simulink model "Arm_Assembly"  (R2025b)
settings: Solver=ode23t  StartTime=0.0  StopTime=10.0  RelTol=1e-3
model workspace: external: MATLAB File C:\Users\kavin\Documents\MATLAB\Arm Project\Arm_Assembly_DataFile.m (data not in the file)
values from neighbouring files (symbols this model uses):
  s = dot(w, u)    [inverse_kinematics.m]
undefined symbols (not defined in the file or in its folder): smiData, X, Y, Z
libraries: sm_lib x36, nesl_utility x14, slpidlib x5
(part 2 of 2)

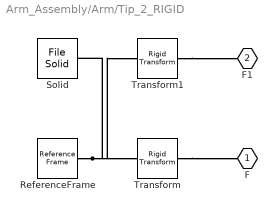
== system Arm_Assembly/Arm/Tip_2_RIGID ==
  ReferenceFrame : sm_lib/Frames and Transforms/Reference Frame
  Solid : sm_lib/Body Elements/File Solid  ExtGeomFileName=Tip_Default_sldprt.STEP  UnitType=FromFile  ExtGeomFileUnits=m  StepReaderType=HEX  ExportConvexHullGeometry=off  InertiaType=Custom  BasedOnType=DensityFromFile  Density=1000  DensityUnits=kg/m^3  Mass=smiData.Solid(7).mass  MassUnits=kg  CenterOfMass=smiData.Solid(7).CoM  CenterOfMassUnits=in  MomentsOfInertia=smiData.Solid(7).MoI  MomentsOfInertiaUnits=kg*in^2  ProductsOfInertia=smiData.Solid(7).PoI  ProductsOfInertiaUnits=kg*in^2  GraphicType=FromGeometry  MarkerShape=Sphere  MarkerSize=10  GraphicVisPropType=SimpleVisualProperties  GraphicDiffuseColor=smiData.Solid(7).color  GraphicOpacity=smiData.Solid(7).opacity  GraphicSpecularColor=[0.5 0.5 0.5 1.0]  GraphicAmbientColor=[0.15 0.15 0.15 1.0]  GraphicEmissiveColor=[0.0 0.0 0.0 1.0]  GraphicShininess=75  DoExposeReferenceFrame=on  SerializedFrames=<Frames/>
  Transform : sm_lib/Frames and Transforms/Rigid Transform  RotationMethod=ArbitraryAxis  FollAlignAxisA=+X  BaseAlignAxisA=+Y  FollAlignAxisB=+Y  BaseAlignAxisB=+Z  RotationStandardAxis=+Z  RotationAngle=smiData.RigidTransform(10).angle  RotationAngleUnits=rad  RotationArbitraryAxis=smiData.RigidTransform(10).axis  RotationSequenceAxes=FollowerAxes  RotationSequence=XYX  RotationSequenceAngles=[0 0 0]  RotationSequenceAnglesUnits=deg  RotationMatrix=[1 0 0;0 1 0;0 0 1]  Quaternion=[1 0 0 0]  TranslationMethod=Cartesian  TranslationCartesianOffset=smiData.RigidTransform(10).translation  TranslationCartesianOffsetUnits=in  TranslationStandardAxis=+Z  TranslationStandardOffset=0  TranslationStandardOffsetUnits=m  TranslationROffset=0  TranslationROffsetUnits=m  TranslationThetaOffset=0  TranslationThetaOffsetUnits=deg  TranslationZOffset=0  TranslationZOffsetUnits=m
  Transform1 : sm_lib/Frames and Transforms/Rigid Transform  RotationMethod=ArbitraryAxis  FollAlignAxisA=+X  BaseAlignAxisA=+Y  FollAlignAxisB=+Y  BaseAlignAxisB=+Z  RotationStandardAxis=+Z  RotationAngle=smiData.RigidTransform(11).angle  RotationAngleUnits=rad  RotationArbitraryAxis=smiData.RigidTransform(11).axis  RotationSequenceAxes=FollowerAxes  RotationSequence=XYX  RotationSequenceAngles=[0 0 0]  RotationSequenceAnglesUnits=deg  RotationMatrix=[1 0 0;0 1 0;0 0 1]  Quaternion=[1 0 0 0]  TranslationMethod=Cartesian  TranslationCartesianOffset=smiData.RigidTransform(11).translation  TranslationCartesianOffsetUnits=in  TranslationStandardAxis=+Z  TranslationStandardOffset=0  TranslationStandardOffsetUnits=m  TranslationROffset=0  TranslationROffsetUnits=m  TranslationThetaOffset=0  TranslationThetaOffsetUnits=deg  TranslationZOffset=0  TranslationZOffsetUnits=m
  F : PMIOPort  Side=Left
  F1 : PMIOPort  Port=2  Side=Right
  connections:
  Solid/RConn1 -- ReferenceFrame/RConn1 -- Transform/LConn1 -- Transform1/LConn1
  Transform/RConn1 -- F/RConn1
  Transform1/RConn1 -- F1/RConn1

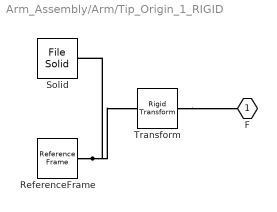
== system Arm_Assembly/Arm/Tip_Origin_1_RIGID ==
  ReferenceFrame : sm_lib/Frames and Transforms/Reference Frame
  Solid : sm_lib/Body Elements/File Solid  ExtGeomFileName=Tip_Origin_Default_sldprt.STEP  UnitType=FromFile  ExtGeomFileUnits=m  StepReaderType=HEX  ExportConvexHullGeometry=off  InertiaType=Custom  BasedOnType=DensityFromFile  Density=1000  DensityUnits=kg/m^3  Mass=smiData.Solid(1).mass  MassUnits=kg  CenterOfMass=smiData.Solid(1).CoM  CenterOfMassUnits=in  MomentsOfInertia=smiData.Solid(1).MoI  MomentsOfInertiaUnits=kg*in^2  ProductsOfInertia=smiData.Solid(1).PoI  ProductsOfInertiaUnits=kg*in^2  GraphicType=FromGeometry  MarkerShape=Sphere  MarkerSize=10  GraphicVisPropType=SimpleVisualProperties  GraphicDiffuseColor=smiData.Solid(1).color  GraphicOpacity=smiData.Solid(1).opacity  GraphicSpecularColor=[0.5 0.5 0.5 1.0]  GraphicAmbientColor=[0.15 0.15 0.15 1.0]  GraphicEmissiveColor=[0.0 0.0 0.0 1.0]  GraphicShininess=75  DoExposeReferenceFrame=on  SerializedFrames=<Frames/>
  Transform : sm_lib/Frames and Transforms/Rigid Transform  RotationMethod=ArbitraryAxis  FollAlignAxisA=+X  BaseAlignAxisA=+Y  FollAlignAxisB=+Y  BaseAlignAxisB=+Z  RotationStandardAxis=+Z  RotationAngle=smiData.RigidTransform(12).angle  RotationAngleUnits=rad  RotationArbitraryAxis=smiData.RigidTransform(12).axis  RotationSequenceAxes=FollowerAxes  RotationSequence=XYX  RotationSequenceAngles=[0 0 0]  RotationSequenceAnglesUnits=deg  RotationMatrix=[1 0 0;0 1 0;0 0 1]  Quaternion=[1 0 0 0]  TranslationMethod=Cartesian  TranslationCartesianOffset=smiData.RigidTransform(12).translation  TranslationCartesianOffsetUnits=in  TranslationStandardAxis=+Z  TranslationStandardOffset=0  TranslationStandardOffsetUnits=m  TranslationROffset=0  TranslationROffsetUnits=m  TranslationThetaOffset=0  TranslationThetaOffsetUnits=deg  TranslationZOffset=0  TranslationZOffsetUnits=m
  F : PMIOPort  Side=Left
  connections:
  Solid/RConn1 -- ReferenceFrame/RConn1 -- Transform/LConn1
  Transform/RConn1 -- F/RConn1

== matlab function Arm_Assembly/MATLAB Function ==
  data: x input; a1 output; y input; z input; r1 input; r2 input; a2 output; a3 output; a4 output; a5 output
function [a1, a2, a3, a4, a5] = inverse_kinematics(x, y, z, r1, r2)
    base = 1.25;
    L1 = 9.1601;
    L2 = 8.0463;
    L3 = 4.7889;
    L4 = 2.0304;
    tip = 2.5245;
    pos = [x, y, z];
    
    r1 = deg2rad(r1);
    r2 = deg2rad(r2);

    tip_v = [sin(r2)*cos(r1), cos(r2), sin(r2)*sin(r1)]; %direction of end
    A = tip_v * tip; %vector of end

    B = pos + A; %target of rest of body
   
    L3 = L3 + L4;
    a1 = atan2(B(3), B(1));
    a1 = a1 + pi - 0.1098;
    l1_v = [0, L1];

    B_t = [sqrt(B(1)*B(1) + B(3)*B(3)), B(2)]; %convert to 2d problem
    %l1 + L2 * <sin(a2), cos(a2)> + L3 * <sin(a2+a3), cos(a2+a3)> = B_t
    
    X_prime = B_t(1);
    Y_prime = B_t(2) - l1_v(2);
    
    robot_system = @(p) [
    L2 * sin(p(1)) + L3 * cos(p(2)) - X_prime; ... % X residual
    L2 * cos(p(1)) + L3 * sin(p(2)) - Y_prime      % Y residual
    ];
    
    initial_guess = [pi/2, pi/4];
    options = optimoptions('fsolve', 'Display', 'off', 'Algorithm', 'levenberg-marquardt');

    [angles_sol, fval, exitflag] = fsolve(robot_system, initial_guess, options);
    
    

    theta1 = angles_sol(1);
    theta2 = angles_sol(2) - pi/2 + theta1;
    theta3 = angles_sol(2);
    
    theta1 = wrapToPi(theta1);
    theta2 = wrapToPi(theta2);
    theta3 = wrapToPi(theta3);

    alpha = atan2(B(3),B(1));
    u = [cos(theta3) * cos(alpha), sin(theta3), cos(theta3) * sin(alpha)];
    
    v_target = cross(u, tip_v);
    
    j = [0, 1, 0];

    % 3. Project the global up-axis onto the link's perpendicular plane
    v_ref = j - dot(j, u) * u;
    
    % 4. Normalize the reference vector
    v_norm = norm(v_ref);
    
    if v_norm > 1e-6
        v_ref = v_ref / v_norm; % This is your perfect "pointing up" reference
    end
    
    v_ref_proj = v_ref - dot(v_ref, u) * u;
    v_target_proj = v_target - dot(v_target, u) * u;
    
    % 3. Normalize the projected vectors
    v_ref_proj = v_ref_proj / norm(v_ref_proj);
    v_target_proj = v_target_proj / norm(v_target_proj);
    
    % 4. Determine cosine via dot product
    c = dot(v_ref_proj, v_target_proj);
    
    % 5. Determine sine via cross product scaled along axis u
    w = cross(v_ref_proj, v_target_proj);
    s = dot(w, u);
    
    % 6. Calculate the final signed angle in radians (-pi to pi)
    twist_angle = atan2(s, c);
    
    a4 = pi + twist_angle;

    a2 = theta1;
    a3 = theta2;
    
    ang = acos(dot(u, tip_v));

    a5 = pi/2 - ang;
end
